simulink model "rwa_step_torqueinput_test"  (R2018b)
settings: Solver=FixedStepAuto  StartTime=0.0  StopTime=60  FixedStep=simParams.sample_time_s  RelTol=1e-3
undefined symbols (not defined in the file): simParams
libraries: rwa_assembly_torqueinput_lib x1, torque_2_rpm_lib x1
settings Model: Creator=Taylor  LastModifiedBy=Taylor

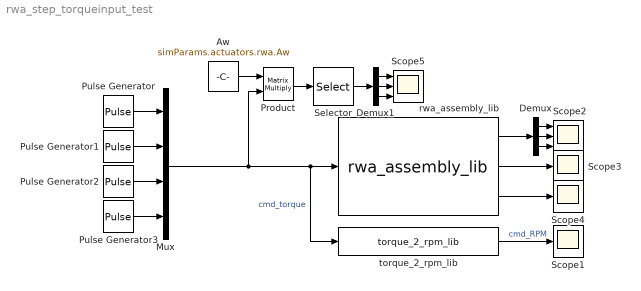
== system rwa_step_torqueinput_test ==
  Aw : Constant  Value=simParams.actuators.rwa.Aw
  Demux : Demux  Outputs=3
  Demux1 : Demux  Outputs=3
  Mux : Mux
  Product : Product  Multiplication=Matrix(*)
  Pulse Generator : DiscretePulseGenerator  PulseType=Time based  Amplitude=3e-3  Period=60  PulseWidth=5  PhaseDelay=10
  Pulse Generator1 : DiscretePulseGenerator  PulseType=Time based  Amplitude=-3e-3  Period=60  PulseWidth=5  PhaseDelay=20
  Pulse Generator2 : DiscretePulseGenerator  PulseType=Time based  Amplitude=3e-3  Period=60  PulseWidth=5  PhaseDelay=30
  Pulse Generator3 : DiscretePulseGenerator  PulseType=Time based  Amplitude=-3e-3  Period=60  PulseWidth=5  PhaseDelay=40
  Scope1 : Scope
  Scope2 : Scope  NumInputPorts=3
  Scope3 : Scope
  Scope4 : Scope
  Scope5 : Scope  NumInputPorts=3
  Selector : Selector  InputPortWidth=4  IndexOptions=Index vector (dialog)  Indices=[1 2 3]  OutputSizes=1
  rwa_assembly_lib : rwa_assembly_torqueinput_lib/rwa_assembly_lib  SystemSampleTime=-1
  torque_2_rpm_lib : torque_2_rpm_lib/torque_2_rpm_lib  SystemSampleTime=-1
  wires:
  Pulse Generator1/1 -> Mux/2
  Pulse Generator3/1 -> Mux/4
  Pulse Generator2/1 -> Mux/3
  Mux/1 -> torque_2_rpm_lib/1, rwa_assembly_lib/1, Product/2  "cmd_torque"
  Pulse Generator/1 -> Mux/1
  Demux/3 -> Scope2/3
  rwa_assembly_lib/3 -> Scope4/1
  rwa_assembly_lib/2 -> Scope3/1
  Demux/2 -> Scope2/2
  Demux/1 -> Scope2/1
  rwa_assembly_lib/1 -> Demux/1
  Demux1/1 -> Scope5/1
  Aw/1 -> Product/1
  Demux1/3 -> Scope5/3
  Selector/1 -> Demux1/1
  Demux1/2 -> Scope5/2
  Product/1 -> Selector/1
  torque_2_rpm_lib/1 -> Scope1/1  "cmd_RPM"
